simulink model "untitled4"  (Simulink 7.7)
settings: Solver=ode45  StartTime=0.0  StopTime=10.0  RelTol=1e-3
libraries: dspxfrm3 x1, dspsrcs4 x1, dspsnks4 x1
settings Model: Creator=ucseo  LastModifiedBy=ucseo

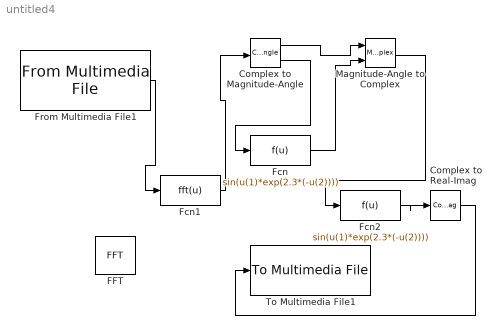
== system untitled4 ==
  Complex to Magnitude-Angle : ComplexToMagnitudeAngle
  Complex to Real-Imag : ComplexToRealImag  Output=Real
  FFT : dspxfrm3/FFT  CompMethod=Table lookup  TableOpt=NEW  TableOptActive=Speed  BitRevOrder=off  InheritFFTLength=on  FFTLength=64  RowConvenienceOn=on  SkipNorm=off  firstCoeffDataTypeStr=Inherit: Same word length as input  firstCoeffLastDataTypeStr=Inherit: Same word length as input  outputMin=[]  outputMax=[]  roundingMode=Floor  overflowMode=off
  Fcn : Fcn  Expr=sin(u(1)*exp(2.3*(-u(2))))
  Fcn1 : Fcn  Expr=fft(u)
  Fcn2 : Fcn  Expr=sin(u(1)*exp(2.3*(-u(2))))
  From Multimedia File1 : dspsrcs4/From Multimedia File  inputFilename=speech_dft.avi  loop=on  numPlays=inf  outputStreams=Video and audio  videoDataType=single  audioDataType=int16  inheritSampleTime=on  userDefinedSampleTime=1/30  noAudioOutput=off  isIntensityVideo=off  fourcc=RGB  colorVideoFormat=Separate color signals  outputEOF=off  dataOrg=Column-major  audioFrameSize=1024  computeAudioFrameSize=off
  Magnitude-Angle to Complex : MagnitudeAngleToComplex
  To Multimedia File1 : dspsnks4/To Multimedia File  outputFilename=output.wav  streamSelection=Audio only  videoCompressor=None (uncompressed)  audioCompressor=MPEG Layer-3  imagePorts=Separate color signals  fileType=WAV  audioDatatype=Determine from input data type  fourcc=RGB
  wires:
  Complex to Magnitude-Angle/2 -> Fcn/1
  Complex to Magnitude-Angle/1 -> Magnitude-Angle to Complex/1
  From Multimedia File1/1 -> Fcn1/1
  Fcn1/1 -> Complex to Magnitude-Angle/1
  Fcn/1 -> Magnitude-Angle to Complex/2
  Magnitude-Angle to Complex/1 -> Fcn2/1
  Fcn2/1 -> Complex to Real-Imag/1
  Complex to Real-Imag/1 -> To Multimedia File1/1
